simulink model "Commands_to_state"  (R2020a)
settings: Solver=VariableStepAuto  StartTime=0.0  StopTime=10.0  RelTol=1e-3
settings Model: Creator=prans  LastModifiedBy=prans

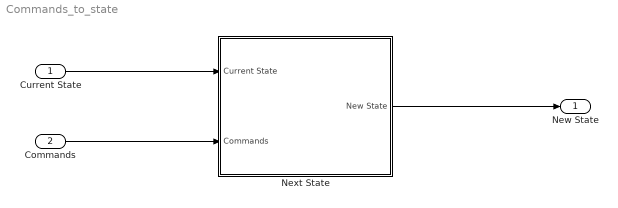
== system Commands_to_state ==
  Current State : Inport
  Commands : Inport  Port=2
  Next State : Subsystem
  New State : Outport
  wires:
  Current State/1 -> Next State/1(Current State)
  Commands/1 -> Next State/2(Commands)
  Next State/1(New State) -> New State/1

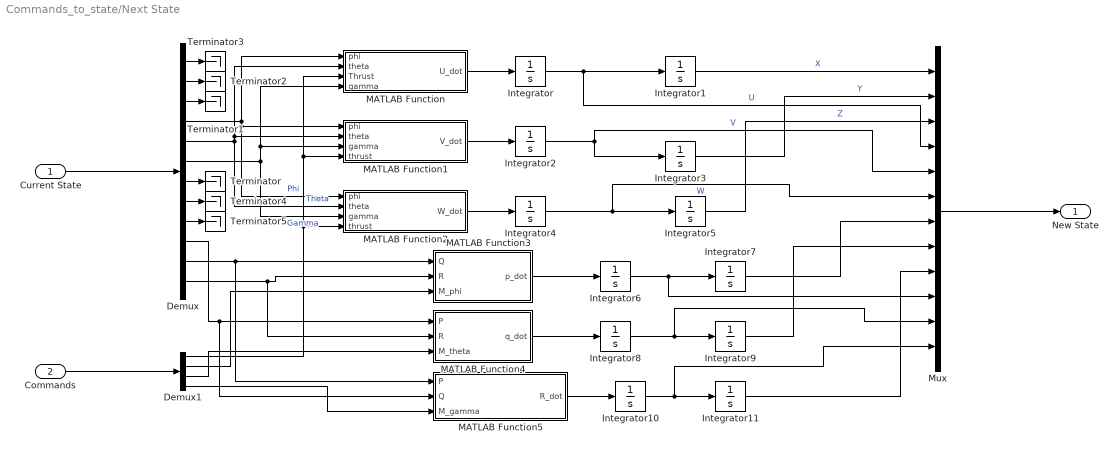
== system Commands_to_state/Next State ==
  Current State : Inport
  Commands : Inport  Port=2
  Demux : Demux  Outputs=12
  Demux1 : Demux
  Integrator{,1..11} (12 alike) : Integrator
  MATLAB Function : MATLAB Function  TreatAsAtomicUnit=on
  MATLAB Function1 : MATLAB Function  TreatAsAtomicUnit=on
  MATLAB Function2 : MATLAB Function  TreatAsAtomicUnit=on
  MATLAB Function3 : MATLAB Function  TreatAsAtomicUnit=on
  MATLAB Function4 : MATLAB Function  TreatAsAtomicUnit=on
  MATLAB Function5 : MATLAB Function  TreatAsAtomicUnit=on
  Mux : Mux  Inputs=12
  Terminator{,1..5} (6 alike) : Terminator
  New State : Outport
  wires:
  MATLAB Function2/1(W_dot) -> Integrator4/1
  Demux/5 -> MATLAB Function1/2(theta), MATLAB Function/2(theta), MATLAB Function2/2(theta)  "Theta"
  Integrator11/1 -> Mux/9
  Demux/10 -> MATLAB Function5/2(Q), MATLAB Function4/1(P)
  Demux1/1 -> MATLAB Function2/4(thrust), MATLAB Function1/4(thrust), MATLAB Function/3(Thrust)
  Integrator6/1 -> Mux/10, Integrator7/1
  Integrator5/1 -> Mux/3  "Z"
  Integrator2/1 -> Integrator3/1, Mux/5  "V"
  MATLAB Function4/1(q_dot) -> Integrator8/1
  Demux/4 -> MATLAB Function2/1(phi), MATLAB Function1/1(phi), MATLAB Function/1(phi)  "Phi"
  Demux/3 -> Terminator1/1
  Integrator7/1 -> Mux/7
  Integrator4/1 -> Mux/6, Integrator5/1  "W"
  Demux/12 -> MATLAB Function4/2(R), MATLAB Function3/2(R)
  Demux/11 -> MATLAB Function5/1(P), MATLAB Function3/1(Q)
  MATLAB Function5/1(R_dot) -> Integrator10/1
  Demux1/3 -> MATLAB Function4/3(M_theta)
  Mux/1 -> New State/1
  Current State/1 -> Demux/1
  Integrator8/1 -> Mux/11, Integrator9/1
  Integrator10/1 -> Mux/12, Integrator11/1
  MATLAB Function1/1(V_dot) -> Integrator2/1
  Integrator1/1 -> Mux/1  "X"
  Demux/6 -> MATLAB Function1/3(gamma), MATLAB Function/4(gamma), MATLAB Function2/3(gamma)  "Gamma"
  Integrator/1 -> Integrator1/1, Mux/4  "U"
  Integrator9/1 -> Mux/8
  MATLAB Function3/1(p_dot) -> Integrator6/1
  Demux1/2 -> MATLAB Function3/3(M_phi)
  Commands/1 -> Demux1/1
  Demux/9 -> Terminator5/1
  Integrator3/1 -> Mux/2  "Y"
  MATLAB Function/1(U_dot) -> Integrator/1
  Demux1/4 -> MATLAB Function5/3(M_gamma)
  Demux/2 -> Terminator2/1
  Demux/1 -> Terminator3/1
  Demux/7 -> Terminator/1
  Demux/8 -> Terminator4/1

== matlab function Commands_to_state/Next State/MATLAB Function1 ==
  data: phi input; theta input; V_dot output; gamma input; thrust input
function V_dot = fcn(phi, theta, gamma, thrust)

V_dot = phi;

== matlab function Commands_to_state/Next State/MATLAB Function ==
  data: phi input; theta input; Thrust input; U_dot output; gamma input
function U_dot = fcn(phi, theta, Thrust, gamma)

y_dot = phi;

== matlab function Commands_to_state/Next State/MATLAB Function2 ==
  data: phi input; theta input; W_dot output; gamma input; thrust input
function W_dot = fcn(phi, theta, gamma, thrust)

V_dot = phi;

== matlab function Commands_to_state/Next State/MATLAB Function3 ==
  data: Q input; R input; p_dot output; M_phi input
function p_dot = fcn(Q, R, M_phi)

y = u;

== matlab function Commands_to_state/Next State/MATLAB Function4 ==
  data: P input; R input; q_dot output; M_theta input
function q_dot = fcn(P, R, M_theta)

y = u;

== matlab function Commands_to_state/Next State/MATLAB Function5 ==
  data: P input; Q input; R_dot output; M_gamma input
function R_dot = fcn(P, Q, M_gamma)

y = u;
